simulink model "LoadFlow58BusNetwork_2024"  (R2024a)
settings: Solver=FixedStepDiscrete  StartTime=0.0  StopTime=4.5  FixedStep=75e-6  RelTol=1e-3  EnableMultiTasking=on
undefined symbols (not defined in the file): D1, D11, Delta
libraries: spsSeriesRLCBranchLib x41, spsLoadFlowBusLib x29, spsDistributedParametersLineLib x19, spsThreePhaseSeriesRLCLoadLib x15, spsThreePhaseTransformerTwoWindingsLib x13, spsThreePhaseParallelRLCLoadLib x11, spsThreePhaseVIMeasurementLib x11, spsSynchronousMachinepuStandardLib x7, spsExcitationSystemLib x7, spsHydraulicTurbineandGovernorLib x7, spsGenericPowerSystemStabilizerLib x7, spsMultiBandPowerSystemStabilizerLib x7
(part 1 of 5)
settings Model: Creator=The MathWorks, Inc.  LastModifiedBy=dilu2
settings SolverCC: AlgebraicLoopSolver=TrustRegion
settings DataIOCC: SaveFormat=StructureWithTime  SaveOutput=off  SaveTime=off  ReturnWorkspaceOutputs=off
settings OptimizationCC: ExpressionDepthLimit=2147483647  LifeSpan=inf
settings DebuggingCC: UnderspecifiedInitializationDetection=Classic  MergeDetectMultiDrivingBlocksExec=none  SolverPrmCheckMsg=warning  FcnCallInpInsideContextMsg=warning  UnconnectedInputMsg=warning  UnconnectedOutputMsg=warning  UnconnectedLineMsg=warning  StateNameClashWarn=warning  SFUnexpectedBacktrackingDiag=warning  SFNoUnconditionalDefaultTransitionDiag=warning  SFExecutionAtInitializationDiag=none  ArithmeticOperatorsInVariantConditions=warning
settings HardwareCC: ProdBitPerPointer=32  ProdBitPerSizeT=32  ProdBitPerPtrDiffT=32  ProdLargestAtomicFloat=None  ProdIntDivRoundTo=Undefined  ProdEndianess=Unspecified  ProdWordSize=32  ProdHWDeviceType=32-bit Generic
settings ModelReferenceCC: EnableRefExpFcnMdlSchedulingChecks=on  PropagateSignalLabelsOutOfModel=off
settings SFSimCC: SimUseLocalCustomCode=off  CustomCodeUndefinedFunction=UseInterfaceOnly
settings RTWCC: RTWUseLocalCustomCode=off  GPUComputeCapability=3.5
settings CodeAppCC: StateflowObjectComments=on
settings GRTTargetCC: TargetLangStandard=C89/C90 (ANSI)  CombineOutputUpdateFcns=off  GRTInterface=on
settings ConfigComp: CovMetricSettings=dw  CovSaveCumulativeToWorkspaceVar=on  CovSaveSingleToWorkspaceVar=on  CovExternalEMLEnable=off  CovSFcnEnable=off
settings SimscapeCC: SimscapeNormalizeSystem=off

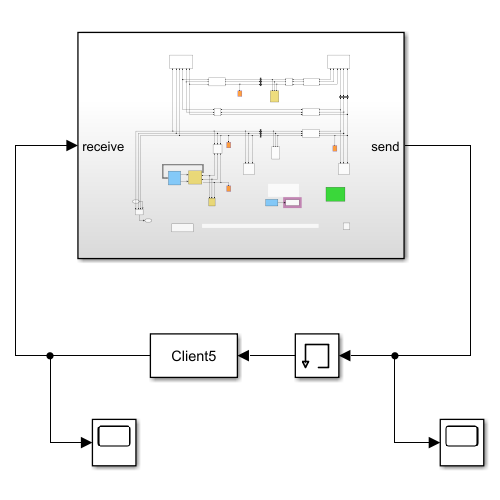
[thumbnail: Simulink's stored preview of the top-level diagram]
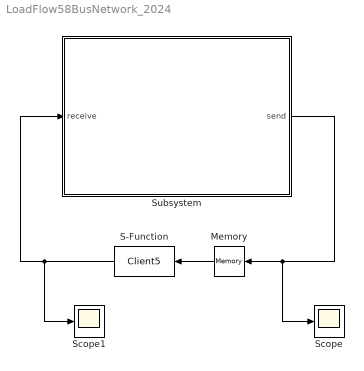
== system LoadFlow58BusNetwork_2024 ==
  Memory : Memory
  S-Function : S-Function  FunctionName=Client5  SFunctionDeploymentMode=off  EnableBusSupport=off
  Scope : Scope
  Scope1 : Scope
  Subsystem : Subsystem
  wires:
  Memory/1 -> S-Function/1
  Subsystem/1(send) -> Scope/1, Memory/1
  S-Function/1 -> Scope1/1, Subsystem/1(receive)

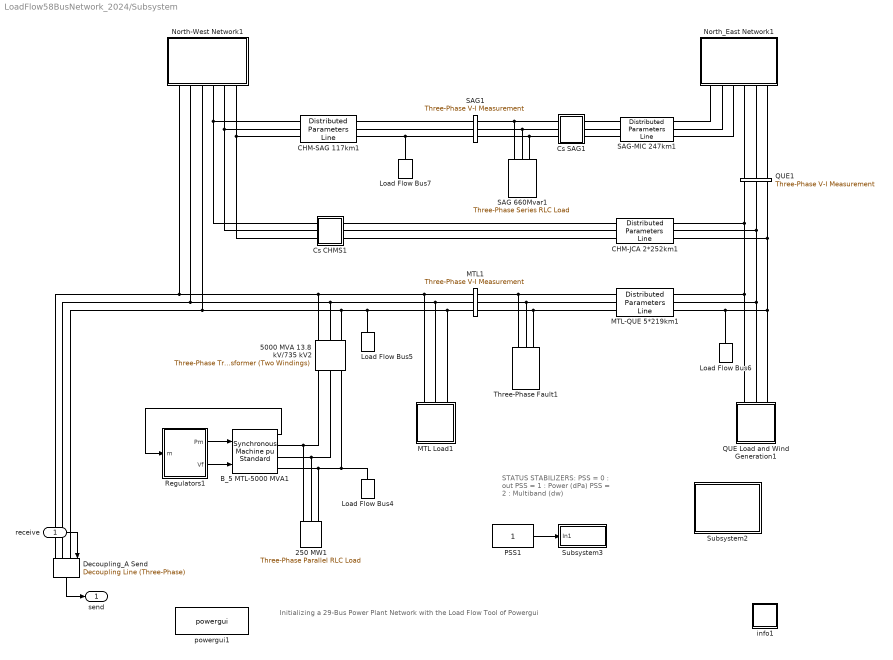
== system LoadFlow58BusNetwork_2024/Subsystem ==
  note: Initializing a 29-Bus Power Plant Network with the Load Flow Tool of Powergui
  note: STATUS STABILIZERS:
      | PSS = 0 :  out
      | PSS = 1 :  Power (dPa)
      | PSS = 2 :  Multiband (dw)
  receive : Inport
  250 MW1 : spsThreePhaseParallelRLCLoadLib/Three-Phase Parallel RLC Load  LConnTagsString=A|B|C  Configuration=Y (grounded)  NominalVoltage=(13800)*1  Vabc=[1e3 1e3 1e3]  Vabcp=[1e3 1e3 1e3]  NominalFrequency=60  UnbalancedPower=off  ActivePower=250000000  InductivePower=0  CapacitivePower=0  Pabc=[10e3 9e3 11e3]  QLabc=[100 90 110]  QCabc=[100 90 110]  Pabcp=[10e3 9e3 11e3]  QLabcp=[100 90 110]  QCabcp=[100 90 110]  Measurements=None  LoadType=constant PQ
  5000 MVA 13.8 kV/735 kV2 : spsThreePhaseTransformerTwoWindingsLib/Three-Phase Transformer (Two Windings)  Winding1Connection=Delta (D1)  Winding2Connection=Yg  CoreType=Three single-phase transformers  SetSaturation=off  Hysteresis=off  DataFile='basic_model'  SetInitialFlux=off  Measurements=None  UNITS=pu  NominalPower=[ 5000e6 60 ]  Winding1="[ 13.8e3 0.002  0.0]"  Winding2=[ 735e3 0.002 0.12]  Rm=500  Lm=500  L0=0.5  Saturation="[ 0,0  ;  0.005,1.2  ;  1.0,1.4 ]"  InitialFluxes=[ 0.8 , -0.8 , 0.7 ]  BreakLoop=off  DiscreteSolver=Trapezoidal iterative  DataType=off  TransfoNumber=0
  B_5 MTL-5000 MVA1 : spsSynchronousMachinepuStandardLib/Synchronous Machine pu Standard  PresetModel=No  MechanicalLoad=Mechanical power Pm  ShowDetailedParameters=on  RotorType=Salient-pole  Units=per unit standard parameters  MeasurementBus=off  NominalParameters="[5000E6  13800   60 ]"  Reactances1=[ 31 32 33 34 35 36 37 ]  Reactances2=[ 1.305, 0.296, 0.252, 0.474, 0.243, 0.18 ]  dAxisTimeConstants=Short-circuit  qAxisTimeConstants=Open-circuit  TimeConstants1=[]  TimeConstants2=[]  TimeConstants3=[]  TimeConstants4=[]  TimeConstants5=[ 1.01, 0.053, 0.1 ]  TimeConstants6=[]  TimeConstants7=[]  TimeConstants8=[]  StatorResistance=2.8544e-3  Mechanical="[ 3.7 0  32]"  PolePairs=32  InitialConditions=[0 -113.876 0.904539 0.904539 0.904539 -42.1129 -162.113 77.8871 1.28555]  SetSaturation=off  Saturation=[0.6404,0.7127,0.8441,0.9214,0.9956,1.082,1.19,1.316,1.457;0.7,0.7698,0.8872,0.9466,0.9969,1.046,1.1,1.151,1.201]  LoadFlowParameters=[1 4000000000 0 0 0]  TsPowergui=0  TsBlock=-1  IterativeModel=Trapezoidal non iterative  IterativeDiscreteModel=Trapezoidal non iterative  BusType=PV  Pref=4500000000  Qref=0  Qmin=-Inf  Qmax=Inf  PLF=0  QLF=0
  CHM-JCA 2*252km1 : spsDistributedParametersLineLib/Distributed Parameters Line  Phases=3  Length=252  Frequency=60  Resistance="[0.01273  0.3864]/2"  Inductance="[0.9337e-3  4.1264e-3]/2"  Capacitance=[12.74e-9 7.751e-9]*2  x1=[-0.0015 2.08314728731826e-08 15714.262594831 -742648.807936676;-0.001425 2.08441228975103e-08 36703.0761534446 -741907.711972178;-0.00135 2.08401104489196e-08 57662.549834557 -740573.546334299;-0.001275 2.08194387349004e-08 78575.9289555982 -738647.377534635;-0.0012 2.07821242801046e-08 99426.4956812844 -736130.745323054;-0.001125 2.07281969131365e-08 120197.582387599 -733025.66145684;-0.00105 2.0657699742708e-08 140872.584985638 -729334.608092525;-0.000975 2.05706891231786e-08 161434.976194663 -725060.535801696;-0.0009 2.04672346095063e-08 181868.318753755 -720206.861212344;-0.000825 2.03474189016463e-08 202156.278561514 -714777.464277674;-0.00075 2.02113377784423e-08 222282.637733286 -708776.685174523;-0.000675 2.0059100021062e-08 242231.307565492 -702209.32083389;-0.0006 1.98908273260395e-08 261986.341396694 -695080.621106345;-0.000525 1.97066542079923e-08 281531.947355108 -687396.284565378;-0.00045 1.95067278920932e-08 300852.50098239 -679162.453952045;-0.000375 1.92912081963801e-08 319932.557723585 -670385.711264557;-0.0003 1.90602674040002e-08 338756.865273267 -661073.072496729;-0.000225 1.88140901254894e-08 357310.375768004 -651231.982029504;-0.00015 1.85528731511975e-08 375578.257815384 -640870.306680029;-7.5e-05 1.82768252939771e-08 393545.908350007 -629996.329413038]  x2=[-0.0015 1.40076837789875e-08 -209700.603633346 -700128.672634885;-0.001425 1.39707979514796e-08 -189823.746323601 -705777.196573694;-0.00135 1.39227440818497e-08 -169795.146815445 -710861.533020316;-0.001275 1.38635605836259e-08 -149630.815664878 -715377.617633987;-0.0012 1.37932947671911e-08 -129346.871929697 -719321.840325766;-0.001125 1.37120028019639e-08 -108959.530284169 -722691.048144382;-0.00105 1.36197496714975e-08 -88485.0880572684 -725482.547796656;-0.000975 1.35166091215329e-08 -67939.9122048419 -727694.107800476;-0.0009 1.34026636010476e-08 -47340.4262261144 -729323.960268613;-0.000825 1.32780041963472e-08 -26703.0970349947 -730370.802321943;-0.00075 1.31427305582526e-08 -6044.42179667621 -730833.797130944;-0.000675 1.29969508224402e-08 14619.0852599438 -730712.574584651;-0.0006 1.28407815230003e-08 35270.9060434865 -730007.231586512;-0.000525 1.26743474992815e-08 55894.531804401 -728718.331976929;-0.00045 1.24977817960958e-08 76473.4763318061 -726846.906082527;-0.000375 1.23112255573648e-08 96991.2891323149 -724394.449892533;-0.0003 1.21148279132913e-08 117431.568580308 -721362.923862902;-0.000225 1.1908745861147e-08 137777.975029141 -717754.751349158;-0.00015 1.16931441397712e-08 158014.24387281 -713572.816669202;-7.5e-05 1.14681950978812e-08 178124.198547625 -708820.46279763]  x3=[-0.0015 5.29913482848101e-11 0.894999888004861 -284.908126309882;-0.001425 5.24485107921031e-11 8.94952227191277 -284.768519995041;-0.00135 5.18637467623581e-11 16.9968905446488 -284.40127408242;-0.001275 5.12375236469932e-11 25.0306717631445 -283.806682142784;-0.0012 5.05703420391853e-11 33.0444438456149 -282.98521948383;-0.001125 4.98627352737034e-11 41.0318007052721 -281.937542770241;-0.00105 4.91152690005692e-11 48.9863573712531 -280.664489498749;-0.000975 4.83285407328847e-11 56.901755092668 -279.167077328663;-0.0009 4.75031793691899e-11 64.7716664216877 -277.44650326836;-0.000825 4.66398446907303e-11 72.5898002716097 -275.504142718419;-0.00075 4.57392268340385e-11 80.3499069458558 -273.341548372142;-0.000675 4.48020457392492e-11 88.0457831338842 -270.960448974363;-0.0006 4.38290505745903e-11 95.6712768700209 -268.362747939508;-0.000525 4.2821019137509e-11 103.220292451247 -265.550521830038;-0.00045 4.17787572329127e-11 110.686795310012 -262.526018696476;-0.000375 4.07030980290208e-11 118.06481683817 -259.291656280351;-0.0003 3.95949013913429e-11 125.3484591582 -255.850020081491;-0.000225 3.8455053195315e-11 132.531899837875 -252.203861291214;-0.00015 3.72844646181448e-11 139.609396544626 -248.356094593069;-7.5e-05 3.60840714104303e-11 146.575291635874 -244.309795832883]  x4=[-0.0015 3.38337818505227e-11 -3172.8334199357 -10043.3125795465;-0.001425 3.4961387413953e-11 -2887.63550825271 -10128.9965094924;-0.00135 3.60610453792117e-11 -2600.12926492673 -10206.5834746075;-0.001275 3.71318766965467e-11 -2310.54451804968 -10276.011453059;-0.0012 3.81730253597873e-11 -2019.11275723742 -10337.2249451831;-0.001125 3.91836590906222e-11 -1726.06694858048 -10390.1750178508;-0.00105 4.01629700039101e-11 -1431.64134841455 -10434.8193435843;-0.000975 4.1110175253491e-11 -1136.07131605956 -10471.1222343927;-0.0009 4.20245176579809e-11 -839.593125676973 -10499.0546703004;-0.000825 4.29052663060518e-11 -542.44377739593 -10518.5943225456;-0.00075 4.37517171407102e-11 -244.860807858905 -10529.7255714292;-0.000675 4.456319352211e-11 52.9178996614269 -10532.4395188013;-0.0006 4.5339046768448e-11 350.65430542244 -10526.7339951737;-0.000525 4.607865667451e-11 648.110403496889 -10512.6135614548;-0.00045 4.67814320074534e-11 945.048412031206 -10490.0895053033;-0.000375 4.744681097943e-11 1241.23096332467 -10459.179832105;-0.0003 4.80742616966702e-11 1536.42129357752 -10419.9092505798;-0.000225 4.86632825846709e-11 1830.38343215632 -10372.3091530295;-0.00015 4.92134027891467e-11 2122.88239022526 -10316.417590244;-7.5e-05 4.97241825524231e-11 2413.68434859265 -10252.2792410834]  x5=0.00142516474882927  V1=ones(3,3)  V2=ones(3,3)  I1=ones(3,3)  I2=ones(3,3)  nHarmo=1  Measurements=None  Decoupling=on  VsMag0=[606505.937088385 606505.59619374 606505.952336152]  VrMag0=[596743.737336323 596743.911083336 596743.706580344]  VsAngle0=[3.61218308623149 -116.387796657602 123.612221103661]  VrAngle0=[-14.273856882167 -134.273869923453 105.726122150021]  IsMag0=[234.023435046632 234.012623108715 234.010085805107]  IrMag0=[8650.9003206612 8650.90619032986 8650.91364627862]  IsAngle0=[2.58186505632488 -117.420380634369 122.583034804954]  IrAngle0=[-15.1321830152099 -135.132103549669 104.867823050539]
      settings: AttributesFormatString=\n  LibrarySourceBlock=sps_lib/Power Grid Elements/Distributed Parameters Line
  CHM-SAG 117km1 : spsDistributedParametersLineLib/Distributed Parameters Line  Phases=3  Length=117  Frequency=60  Resistance="[0.01273  0.3864]"  Inductance="[0.9337e-3  4.1264e-3]"  Capacitance=[12.74e-9 7.751e-9]  x1=[-0.000675 1.91802413039641e-08 161384.253868462 -730188.013921057;-0.0006 1.90228604750691e-08 181962.578167363 -725333.731757154;-0.000525 1.88502730625698e-08 202395.444365398 -719899.628906063;-0.00045 1.86626170302032e-08 222666.518741962 -713890.049306458;-0.000375 1.84600423873302e-08 242759.596910355 -707309.796924322;-0.0003 1.82427110690209e-08 262658.616771325 -700164.131912727;-0.000225 1.80107968066059e-08 282347.671352859 -692458.766406951;-0.00015 1.77644849887981e-08 301811.021525978 -684199.859958284;-7.5e-05 1.7503972513496e-08 321033.108586353 -675394.014610176]  x2=[-0.000675 1.32644576582055e-08 211241.020698699 -709610.354234679;-0.0006 1.31314025060213e-08 231217.678579178 -703354.834381429;-0.000525 1.29878503115909e-08 251009.504585149 -696537.063435265;-0.00045 1.28339158283422e-08 270600.67743373 -689162.491417966;-0.000375 1.26697221091458e-08 289975.536241099 -681237.013449566;-0.0003 1.24954004079486e-08 309118.593041571 -672766.965035891;-0.000225 1.23110900748514e-08 328014.54516844 -663759.117004046;-0.00015 1.21169384447143e-08 346648.287486691 -654220.670089923;-7.5e-05 1.19131007193799e-08 365004.924467822 -644159.249182042]  x3=[-0.000675 1.53791884966281e-11 931.801693491258 -3923.77003572315;-0.0006 1.43946793528256e-11 1042.35686429523 -3895.85908672161;-0.000525 1.33986633225944e-11 1152.07879097047 -3864.83384757478;-0.00045 1.23919366059096e-11 1260.87976348761 -3830.71911938414;-0.000375 1.1375303964705e-11 1368.67280801392 -3793.54217294144;-0.0003 1.0349578079559e-11 1475.37175643891 -3753.33272692882;-0.000225 9.31557890005e-12 1580.89131525574 -3710.12292416222;-0.00015 8.27413298930147e-12 1685.14713374361 -3663.94730589682;-7.5e-05 7.22607286323979e-12 1788.05587139637 -3614.84278421537]  x4=[-0.000675 2.92162426308819e-11 34.7429415929704 -1477.32347167481;-0.0006 2.99900814486756e-11 76.4934319414226 -1475.75088744197;-0.000525 3.07399466542229e-11 118.18277461077 -1472.99861052946;-0.00045 3.14652388167517e-11 159.77764377835 -1469.06884106533;-0.000375 3.21653781488047e-11 201.244789142174 -1463.96472044716;-0.0003 3.28398049697123e-11 242.551062500706 -1457.69032883087;-0.000225 3.34879801529931e-11 283.663444251031 -1450.25068186913;-0.00015 3.41093855573228e-11 324.549069784217 -1441.65172670188;-7.5e-05 3.4703524440729e-11 365.175255756786 -1431.90033720231]  x5=0.000661683633385019  V1=ones(3,3)  V2=ones(3,3)  I1=ones(3,3)  I2=ones(3,3)  nHarmo=1  Measurements=None  Decoupling=on  VsMag0=[610584.183721716 610584.009535667 610584.14443005]  VrMag0=[604521.569069134 604521.776249714 604521.565003261]  VsAngle0=[-2.95698942544824 -122.956984245967 117.043027319659]  VrAngle0=[1.15752648646476 -118.842485295541 121.157503589918]  IsMag0=[3301.92473587884 3301.9203040404 3301.91445622792]  IrMag0=[1209.87683704248 1209.87940955586 1209.88665322207]  IsAngle0=[-2.06102029188923 -122.061181862043 117.93896552265]  IrAngle0=[-14.0730509971364 -134.07258455703 105.92707671982]
      settings: AttributesFormatString=\n  LibrarySourceBlock=sps_lib/Power Grid Elements/Distributed Parameters Line
  Cs CHMS1 : Subsystem  mask{Xc=33/2}
      mask prompts: Xc "Condensator Reactance at  60Hz  (ohm):"
      mask help: Series Compensation
      mask init:
      | Cs=1/Xc/(2*pi*60);
      mask Display: disp('Cs')
  Cs SAG1 : Subsystem  mask{Xc=22}
      mask prompts: Xc "Condensator Reactance at  60Hz  (ohm):"
      mask help: Series Compensation
      mask init:
      | Cs=1/Xc/(2*pi*60);
      mask Display: disp('Cs')
  Decoupling_A Send : spsDecouplingLineThreePhaseLib/Decoupling Line (Three-Phase)  Length=252  Frequency=60  Resistance="[0.01273  0.3864]/2"  Inductance="[0.9337e-3  4.1264e-3]/2"  Capacitance=[12.74e-9 7.751e-9]*2  VsMag0=[520613.013363934 520613.032750504 520613.042981031]  VsAngle0=[95.9069967092205 -144.093005822696 -24.0930027089948]  IhsMag0=[3886.83215054359 3886.83229528369 3886.83237166141]  IhsAngle0=[86.4922430478757 -153.50775948403 -33.5077563702981]  ShowPorts=on  ConnectorID=T34_3229_1960624034510_S
      settings: LibrarySourceBlock=|
      | sps_lib/Power Grid Elements/Decoupling Line
      | (Three-Phase)
  Load Flow Bus4 : spsLoadFlowBusLib/Load Flow Bus  LConnTagsString=a  Phases=single  Connectors=on one side  ID=MTL_13.8  Vbase=13.8e3  Vref=1  Vangle=0  VLF=1  VLFb=1  VLFc=1  angleLF=-47.86  angleLFb=0  angleLFc=0
      settings: AttributesFormatString=%<ID>\n%<Vbase>V\n%<VLF>pu\n%<angleLF>deg.
  Load Flow Bus5 : spsLoadFlowBusLib/Load Flow Bus  LConnTagsString=a  Phases=single  Connectors=on one side  ID=MTL7  Vbase=735e3  Vref=1  Vangle=0  VLF=1.013  VLFb=1  VLFc=1  angleLF=-23.64  angleLFb=0  angleLFc=0
      settings: AttributesFormatString=%<ID>\n%<Vbase>V\n%<VLF>pu\n%<angleLF>deg.
  Load Flow Bus6 : spsLoadFlowBusLib/Load Flow Bus  LConnTagsString=a  Phases=single  Connectors=on one side  ID=QUE7  Vbase=735e3  Vref=1  Vangle=0  VLF=1.023  VLFb=1  VLFc=1  angleLF=-14.99  angleLFb=0  angleLFc=0
      settings: AttributesFormatString=%<ID>\n%<Vbase>V\n%<VLF>pu\n%<angleLF>deg.
  Load Flow Bus7 : spsLoadFlowBusLib/Load Flow Bus  LConnTagsString=a  Phases=single  Connectors=on one side  ID=SAG7  Vbase=735e3  Vref=1  Vangle=0  VLF=1.036  VLFb=1  VLFc=1  angleLF=-0.1653  angleLFb=0  angleLFc=0
      settings: AttributesFormatString=%<ID>\n%<Vbase>V\n%<VLF>pu\n%<angleLF>deg.
  MTL Load1 : Subsystem
  MTL-QUE 5*219km1 : spsDistributedParametersLineLib/Distributed Parameters Line  Phases=3  Length=219  Frequency=60  Resistance="[0.01273  0.3864]/5"  Inductance="[0.9337e-3  4.1264e-3]/5"  Capacitance=[12.74e-9 7.751e-9]*5  x1=[-0.001275 8.74149343994407e-08 0 0;-0.0012 8.73707129290097e-08 0 0;-0.001125 8.72566486474799e-08 0 0;-0.00105 8.70728327360928e-08 0 0;-0.000975 8.68194121344755e-08 0 0;-0.0009 8.64965894231794e-08 0 0;-0.000825 8.61046226617407e-08 -143097.879675133 -713663.77653503;-0.00075 8.56438251823911e-08 -122864.998636676 -717423.987747158;-0.000675 8.51145653395851e-08 -102533.901198206 -720610.701200436;-0.0006 8.45172662155432e-08 -82120.8397279397 -723221.369484888;-0.000525 8.38524052820461e-08 -61642.1321148858 -725253.905672232;-0.00045 8.31205140187514e-08 -41114.1487245756 -726706.684984138;-0.000375 8.23221774883366e-08 -20553.2993128425 -727578.546091053;-0.0003 8.14580338688091e-08 23.980091885227 -727868.792040548;-0.000225 8.05287739433567e-08 20601.2403272944 -727577.190814451;-0.00015 7.95351405481455e-08 41162.0322463955 -726703.975514322;-7.5e-05 7.84779279785086e-08 61689.9198667191 -725249.844175111]  x2=[-0.001275 1.38635605836259e-08 0 0;-0.0012 1.37932947671911e-08 0 0;-0.001125 1.37120028019639e-08 0 0;-0.00105 1.36197496714975e-08 0 0;-0.000975 1.35166091215329e-08 0 0;-0.0009 1.34026636010476e-08 0 0;-0.000825 1.32780041963472e-08 -26703.0970349947 -730370.802321943;-0.00075 1.31427305582526e-08 -6044.42179667621 -730833.797130944;-0.000675 1.29969508224402e-08 14619.0852599438 -730712.574584651;-0.0006 1.28407815230003e-08 35270.9060434865 -730007.231586512;-0.000525 1.26743474992815e-08 55894.531804401 -728718.331976929;-0.00045 1.24977817960958e-08 76473.4763318061 -726846.906082527;-0.000375 1.23112255573648e-08 96991.2891323149 -724394.449892533;-0.0003 1.21148279132913e-08 117431.568580308 -721362.923862902;-0.000225 1.1908745861147e-08 137777.975029141 -717754.751349158;-0.00015 1.16931441397712e-08 158014.24387281 -713572.816669202;-7.5e-05 1.14681950978812e-08 178124.198547625 -708820.46279763]  x3=[-0.001275 3.38356403910686e-10 0 0;-0.0012 3.13475237189635e-10 0 0;-0.001125 2.88343483160307e-10 0 0;-0.00105 2.62981231762344e-10 0 0;-0.000975 2.37408757191458e-10 0 0;-0.0009 2.11646501692549e-10 0 0;-0.000825 1.85715059218486e-10 -5323.24056616569 -20344.1866352303;-0.00075 1.59635158967621e-10 -4745.97060123439 -20486.5462812051;-0.000675 1.33427648813176e-10 -4164.90678002025 -20612.5292955374;-0.0006 1.07113478637782e-10 -3580.51359605137 -20722.0349693331;-0.000525 8.07136835864552e-11 -2993.2582042975 -20814.9757654321;-0.00045 5.42493672514307e-11 -2403.6100477335 -20891.277388384;-0.000375 2.77416848022685e-11 -1812.04048207381 -20950.8788438389;-0.0003 1.21182607473737e-12 -1219.0223989779 -20993.7324873053;-0.000225 -2.53190013680163e-11 -625.029848027918 -21019.8040622361;-0.00015 -5.18295891884701e-11 -30.5376577806965 -21029.0727274134;-7.5e-05 -7.8298745228346e-11 563.978943802912 -21021.531073608]  x4=[-0.001275 2.95644055162341e-10 0 0;-0.0012 3.24049227246394e-10 0 0;-0.001125 3.52195359336306e-10 0 0;-0.00105 3.80059951844735e-10 0 0;-0.000975 4.07620730242771e-10 0 0;-0.0009 4.34855662865857e-10 0 0;-0.000825 4.61742978525563e-10 -1592.00824148551 -5672.40977476208;-0.00075 4.8826118391314e-10 -1431.01007071774 -5715.14957068699;-0.000675 5.14389080780944e-10 -1268.86797239464 -5753.32076348981;-0.0006 5.40105782887988e-10 -1105.71156042873 -5786.89283970306;-0.000525 5.65390732696087e-10 -941.671259559369 -5815.83896232268;-0.00045 5.90223717803237e-10 -776.878201093171 -5840.13599226114;-0.000375 6.14584887101101e-10 -611.464118079654 -5859.76450684446;-0.0003 6.3845476664368e-10 -445.561240005859 -5874.70881533841;-0.000225 6.6181427521449e-10 -279.302187094119 -5884.95697149145;-0.00015 6.84644739579792e-10 -112.819864287482 -5890.50078308433;-7.5e-05 7.06927909415689e-10 53.752644992464 -5891.3358184789]  x5=0.00123853603172068  V1=ones(3,3)  V2=ones(3,3)  I1=ones(3,3)  I2=ones(3,3)  nHarmo=1  Measurements=None  Decoupling=on  VsMag0=[594302.518281079 594302.525591473 594302.380387402]  VrMag0=[596743.737336323 596743.911083336 596743.706580344]  VsAngle0=[-23.5181046799965 -143.51812043764 96.4818868308265]  VrAngle0=[-14.273856882167 -134.273869923453 105.726122150021]  IsMag0=[17258.8321886677 17258.8369567323 17258.821705247]  IrMag0=[4835.28137561733 4835.27973459469 4835.28879561644]  IsAngle0=[-26.8431826212202 -146.843231946901 93.1567790076211]  IrAngle0=[-27.8572964468753 -147.857183694816 92.1427767692567]
      settings: AttributesFormatString=\n  LibrarySourceBlock=sps_lib/Power Grid Elements/Distributed Parameters Line
  MTL1 : spsThreePhaseVIMeasurementLib/Three-Phase V-I Measurement  VoltageMeasurement=phase-to-ground  SetLabelV=on  LabelV=Vabc_MTL7_1  Vpu=on  VpuLL=off  CurrentMeasurement=no  SetLabelI=off  LabelI=A1  Ipu=off  Pbase=100e6  Vbase=735e3  OutputType=Magnitude  PhasorSimulation=off  PSBequivalent=0
  North-West Network1 : Subsystem
  North_East Network1 : Subsystem
  PSS1 : Constant
  QUE Load and Wind Generation1 : Subsystem
  QUE1 : spsThreePhaseVIMeasurementLib/Three-Phase V-I Measurement  VoltageMeasurement=no  SetLabelV=on  LabelV=Vabc_QUE7  Vpu=on  VpuLL=off  CurrentMeasurement=no  SetLabelI=off  LabelI=A1  Ipu=off  Pbase=100e6  Vbase=735e3  OutputType=Magnitude  PhasorSimulation=off  PSBequivalent=0
  Regulators1 : Subsystem
  SAG 660Mvar1 : spsThreePhaseSeriesRLCLoadLib/Three-Phase Series RLC Load  LConnTagsString=A|B|C  Configuration=Y (grounded)  NominalVoltage=735e3  Vabc=[1e3 1e3 1e3]  Vabcp=[1e3 1e3 1e3]  NominalFrequency=60  UnbalancedPower=off  ActivePower=2200000  InductivePower=660e6  CapacitivePower=0  Pabc=[10e3 9e3 11e3]  QLabc=[100 90 110]  QCabc=[100 90 110]  Pabcp=[10e3 9e3 11e3]  QLabcp=[100 90 110]  QCabcp=[100 90 110]  Measurements=None  LoadType=constant Z
  SAG-MIC 247km1 : spsDistributedParametersLineLib/Distributed Parameters Line  Phases=3  Length=247  Frequency=60  Resistance="[0.01273  0.3864]/1"  Inductance="[0.9337e-3  4.1264e-3]/1"  Capacitance=[12.74e-9 7.751e-9]*1  x1=[-0.001425 1.47124469074144e-08 -23892.3616667774 -729222.084147013;-0.00135 1.46899929834646e-08 -3267.28940140246 -729606.070163554;-0.001275 1.46557961038881e-08 17360.3946851287 -729406.820250953;-0.0012 1.46098836051474e-08 37974.2011377716 -728624.493686542;-0.001125 1.45522921889915e-08 58557.6515950497 -727259.715850207;-0.00105 1.44830678931173e-08 79094.2919616048 -725313.577724468;-0.000975 1.44022660543676e-08 99567.7055613491 -722787.635022366;-0.0009 1.43099512644962e-08 119961.526260705 -719683.906943849;-0.000825 1.42061973185335e-08 140259.45155144 -716004.874561653;-0.00075 1.40910871557964e-08 160445.255582647 -711753.478837975;-0.000675 1.39647127935879e-08 180502.802131436 -706933.118273508;-0.0006 1.38271752536395e-08 200416.057501987 -701547.646190732;-0.000525 1.36785844813562e-08 220169.103342639 -695601.36765363;-0.00045 1.35190592579279e-08 239746.149370779 -689099.036026284;-0.000375 1.33487271053773e-08 259131.545995351 -682045.849173106;-0.0003 1.3167724184621e-08 278309.7968269 -674447.445303752;-0.000225 1.29761951866245e-08 297265.571065148 -666309.898466013;-0.00015 1.27742932167383e-08 315983.715754203 -657639.713690325;-7.5e-05 1.25621796723078e-08 334449.267895597 -648443.821789737]  x2=[-0.001425 4.75263384881545e-09 88893.3544414114 -739233.912944179;-0.00135 4.71488557756924e-09 109756.40330771 -736425.413361934;-0.001275 4.67336829893249e-09 130531.714584533 -733028.226571933;-0.0012 4.62811520118251e-09 151202.68080592 -729045.068233319;-0.001125 4.57916245895323e-09 171752.777917749 -724479.122421923;-0.00105 4.52654920431781e-09 192165.578486817 -719334.039084965;-0.000975 4.47031749550698e-09 212424.764832674 -713613.931123342;-0.0009 4.41051228328839e-09 232514.142071731 -707323.371103838;-0.000825 4.34718137503364e-09 252417.651063202 -700467.387603885;-0.00075 4.2803753965018e-09 272119.381246533 -693051.461191792;-0.000675 4.21014775136993e-09 291603.583360062 -685081.520045664;-0.0006 4.13655457854304e-09 310854.682030736 -676563.935214511;-0.000525 4.05965470727746e-09 329857.288224832 -667505.515525323;-0.00045 3.97950961015369e-09 348596.211549706 -657913.502140201;-0.000375 3.8961833539361e-09 367056.472396769 -647795.562767882;-0.0003 3.80974254835898e-09 385223.31391595 -637159.785534291;-0.000225 3.72025629287972e-09 403082.213812101 -626014.672517016;-0.00015 3.62779612144176e-09 420618.895953895 -614369.132948876;-7.5e-05 3.53243594529146e-09 437819.341785948 -602232.476096019]  x3=[-0.001425 1.449181420039e-11 -591.222973545874 -3970.47337116317;-0.00135 1.3927631720128e-11 -478.738749485206 -3985.6004368759;-0.001275 1.33523157041689e-11 -365.871828993148 -3997.54147458112;-0.0012 1.27663260513332e-11 -252.71243615902 -4006.28693879599;-0.001125 1.21701311927833e-11 -139.351028870057 -4011.82983853024;-0.00105 1.15642077175673e-11 -25.8782265007565 -4014.16574287462;-0.000975 1.09490399916401e-11 87.6152625268583 -4013.29278454294;-0.0009 1.03251197706695e-11 201.038713254167 -4009.21166136473;-0.000825 9.69294580693383e-12 314.301456710097 -4001.92563572743;-0.00075 9.05302345062717e-12 427.312952390505 -3991.44053196844;-0.000675 8.40586424588999e-12 539.982860634881 -3977.76473171929;-0.0006 7.75198552188868e-12 652.221114842479 -3960.90916720544;-0.000525 7.09190997927053e-12 763.93799347019 -3940.88731250727;-0.00045 6.42616527232481e-12 875.044191754565 -3917.71517278907;-0.000375 5.75528358718402e-12 985.450893100676 -3891.41127150481;-0.0003 5.07980121640243e-12 1095.06984008075 -3861.99663559069;-0.000225 4.40025813025201e-12 1203.81340498579 -3829.49477865661;-0.00015 3.71719754507847e-12 1311.59465987384 -3793.9316821897;-7.5e-05 3.03116548906243e-12 1418.32744605887 -3755.33577478516]  x4=[-0.001425 9.72811966664692e-12 -44.2696955264446 -1445.03567527927;-0.00135 1.03978814794709e-11 -3.40032222034586 -1445.70991618316;-0.001275 1.10593313849332e-11 37.471769251309 -1445.22847870017;-0.0012 1.17119406300998e-11 78.3139063639618 -1443.59174768403;-0.001125 1.23551875291253e-11 119.09344053811 -1440.8010315125;-0.00105 1.29885578802808e-11 159.777773238083 -1436.85856104137;-0.000975 1.36115453769985e-11 200.334382030812 -1431.76748782121;-0.0009 1.42236520126053e-11 240.730846583763 -1425.53188157807;-0.000825 1.48243884784225e-11 280.934874581261 -1418.15672696016;-0.00075 1.54132745549107e-11 320.914327538467 -1409.64791955325;-0.000675 1.59898394955508e-11 360.637246492392 -1400.01226116778;-0.0006 1.65536224031509e-11 400.071877549406 -1389.25745440164;-0.000525 1.71041725982808e-11 439.186697268812 -1377.3920964828;-0.00045 1.76410499795383e-11 477.950437862204 -1364.42567239684;-0.000375 1.81638253753592e-11 516.332112188455 -1350.36854730478;-0.0003 1.86720808870909e-11 554.301038524369 -1335.23195825734;-0.000225 1.91654102230539e-11 591.826865091176 -1319.0280052122;-0.00015 1.96434190233252e-11 628.879594317285 -1301.7696413615;-7.5e-05 2.01057251749837e-11 665.429606817877 -1283.47066277723]  x5=0.00139688767047948  V1=ones(3,3)  V2=ones(3,3)  I1=ones(3,3)  I2=ones(3,3)  nHarmo=1  Measurements=None  Decoupling=on  VsMag0=[595726.858585737 595726.856922626 595726.834929731]  VrMag0=[607930.23167611 607930.976808519 607930.152146887]  VsAngle0=[-1.09657636564089 -121.096578900452 118.903422505478]  VrAngle0=[7.63692875074935 -112.363120449623 127.636843332422]  IsMag0=[3296.72064632886 3296.71771518503 3296.71033953548]  IrMag0=[1187.28543067559 1187.29227239663 1187.29553954474]  IsAngle0=[-7.68926033426767 -127.689437762273 112.310695069139]  IrAngle0=[-0.975042579703497 -120.974669903312 119.024857828983]
      settings: AttributesFormatString=\n  LibrarySourceBlock=sps_lib/Power Grid Elements/Distributed Parameters Line
  SAG1 : spsThreePhaseVIMeasurementLib/Three-Phase V-I Measurement  VoltageMeasurement=no  SetLabelV=on  LabelV=Vabc_SAG7  Vpu=on  VpuLL=off  CurrentMeasurement=no  SetLabelI=off  LabelI=Iabc_SAG7  Ipu=off  Pbase=100e6  Vbase=735e3  OutputType=Magnitude  PhasorSimulation=off  PSBequivalent=0
  Subsystem2 : Subsystem
      mask Display: disp('Display\nWaveforms')
  Subsystem3 : Subsystem
      mask Display: disp('PSS_select')
  Three-Phase Fault1 : spsThreePhaseFaultLib/Three-Phase Fault  InitialStates=0  FaultA=on  FaultB=on  FaultC=on  GroundFault=on  SwitchTimes=[0.2 0.3]  External=off  SwitchStatus=NaN  FaultResistance=0.001  GroundResistance=0.001  SnubberResistance=1e6  SnubberCapacitance=inf  Measurements=None
  info1 : Subsystem
      settings: OpenFcn="showExample(\"simscapeelectricalsps/LoadFlow29BusNetworkExample\")"
      mask Display: disp('?')
  powergui1 : sps_lib/powergui  Priority=1  SimulationMode=Discrete  SampleTime=75e-6  frequency=60  Iterations=50  frequencyindice=60  Pbase=1e+008  ErrMax=0.0001  UnitsV=kV  UnitsW=MW  buscounter=0  FunctionMessages=off  echomessages=off  EnableUseOfTLC=off  CurrentSourceSwitches=off  DisableSnubberDevices=off  DisableRonSwitches=off  DisableVfSwitches=off  DisplayEquations=off  AutomaticDiscreteSolvers=off  SolverType=Tustin/Backward Euler (TBE)  Interpol=off  ExternalGateDelay=off  methode=off  Ts=100  x0status=blocks  SPID=off  SwTol=0  HookPort=off  NonlinearTolerance=1e-4  nMaxIteration=100  ContinueOnMaxIteration=off  RestoreLinks=warning  ResistiveCurrentMeasurement=off  Frange=[0:2:500]  Ylog=off  Xlog=on  ShowGrid=off  save=off  variable=ZData  structure=0  ZoomFFT=off  StartTime=0.0  cycles=1  DisplayStyle=1  fundamental=60  FreqAxis=off  MaxFrequency=1000  frequencyindicesteady=1  RmsSteady=1  display=off
  send : Outport
  wires:
  receive/1 -> Decoupling_A Send/1
  Regulators1/2(Vf) -> B_5 MTL-5000 MVA1/2
  Decoupling_A Send/1 -> send/1
  Regulators1/1(Pm) -> B_5 MTL-5000 MVA1/1
  B_5 MTL-5000 MVA1/1 -> Regulators1/1(m)
  PSS1/1 -> Subsystem3/1(In1)
  connections:
  QUE1/RConn1 -- North_East Network1/LConn4
  MTL-QUE 5*219km1/RConn2 -- QUE1/LConn2 -- CHM-JCA 2*252km1/RConn2 -- QUE Load and Wind Generation1/LConn2
  Load Flow Bus6/LConn1 -- MTL-QUE 5*219km1/RConn3 -- QUE1/LConn3 -- CHM-JCA 2*252km1/RConn3 -- QUE Load and Wind Generation1/LConn3
  SAG1/RConn2 -- SAG 660Mvar1/LConn2 -- Cs SAG1/LConn2
  5000 MVA 13.8 kV/735 kV2/RConn2 -- Decoupling_A Send/LConn2 -- North-West Network1/RConn2 -- MTL1/LConn2 -- MTL Load1/LConn2
  MTL-QUE 5*219km1/LConn2 -- MTL1/RConn2 -- Three-Phase Fault1/LConn2
  CHM-SAG 117km1/RConn3 -- SAG1/LConn3 -- Load Flow Bus7/LConn1
  CHM-SAG 117km1/LConn3 -- North-West Network1/RConn6 -- Cs CHMS1/LConn3
  QUE1/RConn2 -- North_East Network1/LConn5
  5000 MVA 13.8 kV/735 kV2/LConn3 -- 250 MW1/LConn3 -- B_5 MTL-5000 MVA1/RConn3 -- Load Flow Bus4/LConn1
  SAG1/RConn1 -- SAG 660Mvar1/LConn1 -- Cs SAG1/LConn1
  SAG1/RConn3 -- SAG 660Mvar1/LConn3 -- Cs SAG1/LConn3
  SAG-MIC 247km1/RConn3 -- North_East Network1/LConn3
  Cs CHMS1/RConn2 -- CHM-JCA 2*252km1/LConn2
  CHM-SAG 117km1/LConn2 -- North-West Network1/RConn5 -- Cs CHMS1/LConn2
  CHM-SAG 117km1/LConn1 -- North-West Network1/RConn4 -- Cs CHMS1/LConn1
  Cs SAG1/RConn3 -- SAG-MIC 247km1/LConn3
  SAG-MIC 247km1/RConn2 -- North_East Network1/LConn2
  Cs CHMS1/RConn1 -- CHM-JCA 2*252km1/LConn1
  5000 MVA 13.8 kV/735 kV2/RConn3 -- Decoupling_A Send/LConn1 -- North-West Network1/RConn3 -- MTL1/LConn3 -- MTL Load1/LConn3 -- Load Flow Bus5/LConn1
  MTL Load1/LConn1 -- MTL1/LConn1 -- Decoupling_A Send/LConn3 -- North-West Network1/RConn1 -- 5000 MVA 13.8 kV/735 kV2/RConn1
  MTL-QUE 5*219km1/LConn1 -- MTL1/RConn1 -- Three-Phase Fault1/LConn1
  Cs SAG1/RConn1 -- SAG-MIC 247km1/LConn1
  MTL-QUE 5*219km1/RConn1 -- QUE1/LConn1 -- CHM-JCA 2*252km1/RConn1 -- QUE Load and Wind Generation1/LConn1
  Cs CHMS1/RConn3 -- CHM-JCA 2*252km1/LConn3
  Cs SAG1/RConn2 -- SAG-MIC 247km1/LConn2
  SAG1/LConn2 -- CHM-SAG 117km1/RConn2
  QUE1/RConn3 -- North_East Network1/LConn6
  SAG1/LConn1 -- CHM-SAG 117km1/RConn1
  SAG-MIC 247km1/RConn1 -- North_East Network1/LConn1
  250 MW1/LConn1 -- 5000 MVA 13.8 kV/735 kV2/LConn1 -- B_5 MTL-5000 MVA1/RConn1
  250 MW1/LConn2 -- 5000 MVA 13.8 kV/735 kV2/LConn2 -- B_5 MTL-5000 MVA1/RConn2
  MTL-QUE 5*219km1/LConn3 -- MTL1/RConn3 -- Three-Phase Fault1/LConn3

== system LoadFlow58BusNetwork_2024/Subsystem/Cs CHMS1 ==
  note: B
  Ca : spsSeriesRLCBranchLib/Series RLC Branch  LConnTagsString=__new0  RConnTagsString=__new0  BranchType=C  Resistance=1.0  Inductance=1.0  SetiL0=off  InitialCurrent=0  Capacitance=Cs  Setx0=off  InitialVoltage=0  Measurements=None
  Cb : spsSeriesRLCBranchLib/Series RLC Branch  LConnTagsString=__new0  RConnTagsString=__new0  BranchType=C  Resistance=1.0  Inductance=1.0  SetiL0=off  InitialCurrent=0  Capacitance=Cs  Setx0=off  InitialVoltage=0  Measurements=None
  Cc : spsSeriesRLCBranchLib/Series RLC Branch  LConnTagsString=__new0  RConnTagsString=__new0  BranchType=C  Resistance=1.0  Inductance=1.0  SetiL0=off  InitialCurrent=0  Capacitance=Cs  Setx0=off  InitialVoltage=0  Measurements=None
  A : PMIOPort  Side=Left
  B : PMIOPort  Port=2  Side=Left
  C : PMIOPort  Port=3  Side=Left
  "A " : PMIOPort  Port=4  Side=Right
  "B " : PMIOPort  Port=5  Side=Right
  "C " : PMIOPort  Port=6  Side=Right
  connections:
  Cc/RConn1 -- "C "/RConn1
  C/RConn1 -- Cc/LConn1
  Cb/RConn1 -- "B "/RConn1
  B/RConn1 -- Cb/LConn1
  Ca/RConn1 -- "A "/RConn1
  A/RConn1 -- Ca/LConn1

== system LoadFlow58BusNetwork_2024/Subsystem/Cs SAG1 ==
  note: B
  Ca : spsSeriesRLCBranchLib/Series RLC Branch  LConnTagsString=__new0  RConnTagsString=__new0  BranchType=C  Resistance=1.0  Inductance=1.0  SetiL0=off  InitialCurrent=0  Capacitance=Cs  Setx0=off  InitialVoltage=0  Measurements=None
  Cb : spsSeriesRLCBranchLib/Series RLC Branch  LConnTagsString=__new0  RConnTagsString=__new0  BranchType=C  Resistance=1.0  Inductance=1.0  SetiL0=off  InitialCurrent=0  Capacitance=Cs  Setx0=off  InitialVoltage=0  Measurements=None
  Cc : spsSeriesRLCBranchLib/Series RLC Branch  LConnTagsString=__new0  RConnTagsString=__new0  BranchType=C  Resistance=1.0  Inductance=1.0  SetiL0=off  InitialCurrent=0  Capacitance=Cs  Setx0=off  InitialVoltage=0  Measurements=None
  A : PMIOPort  Side=Left
  B : PMIOPort  Port=2  Side=Left
  C : PMIOPort  Port=3  Side=Left
  "A " : PMIOPort  Port=4  Side=Right
  "B " : PMIOPort  Port=5  Side=Right
  "C " : PMIOPort  Port=6  Side=Right
  connections:
  A/RConn1 -- Ca/LConn1
  Ca/RConn1 -- "A "/RConn1
  B/RConn1 -- Cb/LConn1
  Cb/RConn1 -- "B "/RConn1
  C/RConn1 -- Cc/LConn1
  Cc/RConn1 -- "C "/RConn1

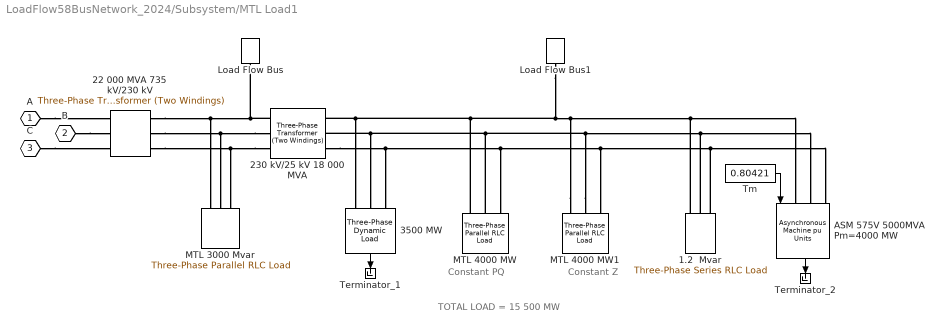
== system LoadFlow58BusNetwork_2024/Subsystem/MTL Load1 ==
  note: Constant PQ
  note: Constant Z
  note: TOTAL LOAD = 15 500 MW
  1.2  Mvar : spsThreePhaseSeriesRLCLoadLib/Three-Phase Series RLC Load  LConnTagsString=A|B|C  Configuration=Y (grounded)  NominalVoltage=25e3  Vabc=[1e3 1e3 1e3]  Vabcp=[1e3 1e3 1e3]  NominalFrequency=60  UnbalancedPower=off  ActivePower=2000e6/50  InductivePower=0  CapacitivePower=2000e6  Pabc=[10e3 9e3 11e3]  QLabc=[100 90 110]  QCabc=[100 90 110]  Pabcp=[10e3 9e3 11e3]  QLabcp=[100 90 110]  QCabcp=[100 90 110]  Measurements=None  LoadType=constant Z
  22 000 MVA 735 kV/230 kV : spsThreePhaseTransformerTwoWindingsLib/Three-Phase Transformer (Two Windings)  Winding1Connection=Yg  Winding2Connection=Delta (D1)  CoreType=Three single-phase transformers  SetSaturation=off  Hysteresis=off  DataFile='basic_model'  SetInitialFlux=off  Measurements=None  UNITS=pu  NominalPower=[ 22000e6 60 ]  Winding1="[ 735e3 0.002  0.12]"  Winding2=[230e3 0.002 0]  Rm=500  Lm=500  L0=0.5  Saturation="[ 0,0  ;  0.005,1.2  ;  1.0,1.4 ]"  InitialFluxes=[ 0.8 , -0.8 , 0.7 ]  BreakLoop=off  DiscreteSolver=Trapezoidal iterative  DataType=off  TransfoNumber=0
  230 kV/25 kV 18 000 MVA : spsThreePhaseTransformerTwoWindingsLib/Three-Phase Transformer (Two Windings)  Winding1Connection=Yg  Winding2Connection=Delta (D1)  CoreType=Three single-phase transformers  SetSaturation=off  Hysteresis=off  DataFile='basic_model'  SetInitialFlux=off  Measurements=None  UNITS=pu  NominalPower=[18000e6 60 ]  Winding1="[ 230e3  0.08/30   0.08 ]"  Winding2="[ 25e3  0.08/30  0.08]"  Rm=500  Lm=500  L0=0.5  Saturation="[ 0,0  ;  0.005,1.2  ;  1.0,1.4 ]"  InitialFluxes=[ 0.8 , -0.8 , 0.7 ]  BreakLoop=off  DiscreteSolver=Trapezoidal iterative  DataType=off  TransfoNumber=0
  3500 MW : spsThreePhaseDynamicLoadLib/Three-Phase Dynamic Load  NominalVoltage=[ 25e3 60 ]  ActiveReactivePowers=[3.5e+09 4.44089e-08]  PositiveSequence=[0.991615 -96.3945]  ExternalControl=off  NpNq="[1.5  2.5]"  TimeConstants="[0  0  0  0]"  MinimumVoltage=0.7  Tfilter=1e-4  LoadFlowParameters=[4,0,0,0,0]
      settings: LibrarySourceBlock=|
      | sps_lib/Passives/Three-Phase
      | Dynamic Load
  ASM 575V 5000MVA Pm=4000 MW : spsAsynchronousMachinepuUnitsLib/Asynchronous Machine pu Units  RotorType=Squirrel-cage  PresetModel=No  MechanicalLoad=Torque Tm  ShowDetailedParameters=on  ReferenceFrame=Rotor  Units=pu  MeasurementBus=off  NominalParameters="[5000e6 25e3  60]"  VoltageRatio=1  Stator=[0.01117 0.04832]  Rotor=[0.006 0.04832]  Cage1=[0.01909 0.0397]  Cage2=[0.01909 0.0397]  Lm=2.424  Mechanical="[1  0   2]"  PolePairs=2  InitialConditions=[0.00523668 0 0.941796 0.941796 0.941796 -125.733 -245.733 -5.73298]  SimulateSaturation=off  Saturation="[0.212,0.4201,0.8125,1.0979,1.4799,2.2457,3.2586,4.5763,6.4763 ;   0.5,0.7,0.9,1,1.1,1.2 ,1.3,1.4,1.5]"  LoadFlowParameters=0  TsPowergui=0  TsBlock=-1  IterativeModel=Trapezoidal non iterative  IterativeDiscreteModel=Trapezoidal non iterative  Pmec=4000000000
      settings: LibrarySourceBlock=|
      | sps_lib/Electrical Machines/Asynchronous Machine
      | pu Units
  Load Flow Bus : spsLoadFlowBusLib/Load Flow Bus  LConnTagsString=a  Phases=single  Connectors=on one side  ID=MTL2  Vbase=230e3  Vref=1  Vangle=0  VLF=1.009  VLFb=1  VLFc=1  angleLF=-58.45  angleLFb=0  angleLFc=0
      settings: AttributesFormatString=%<ID>\n%<Vbase>V\n%<VLF>pu\n%<angleLF>deg.
  Load Flow Bus1 : spsLoadFlowBusLib/Load Flow Bus  LConnTagsString=a  Phases=single  Connectors=on one side  ID=MTL_25  Vbase=25e3  Vref=1  Vangle=0  VLF=0.9916  VLFb=1  VLFc=1  angleLF=-96.39  angleLFb=0  angleLFc=0
      settings: AttributesFormatString=%<ID>\n%<Vbase>V\n%<VLF>pu\n%<angleLF>deg.
  MTL 3000 Mvar : spsThreePhaseParallelRLCLoadLib/Three-Phase Parallel RLC Load  LConnTagsString=A|B|C  Configuration=Y (grounded)  NominalVoltage=230e3  Vabc=[1e3 1e3 1e3]  Vabcp=[1e3 1e3 1e3]  NominalFrequency=60  UnbalancedPower=off  ActivePower=0  InductivePower=0  CapacitivePower=3000e6  Pabc=[10e3 9e3 11e3]  QLabc=[100 90 110]  QCabc=[100 90 110]  Pabcp=[10e3 9e3 11e3]  QLabcp=[100 90 110]  QCabcp=[100 90 110]  Measurements=None  LoadType=constant Z
  MTL 4000 MW : spsThreePhaseParallelRLCLoadLib/Three-Phase Parallel RLC Load  LConnTagsString=A|B|C  Configuration=Y (grounded)  NominalVoltage=(25000)*0.991615  Vabc=[1e3 1e3 1e3]  Vabcp=[1e3 1e3 1e3]  NominalFrequency=60  UnbalancedPower=off  ActivePower=4000000000  InductivePower=0  CapacitivePower=0  Pabc=[10e3 9e3 11e3]  QLabc=[100 90 110]  QCabc=[100 90 110]  Pabcp=[10e3 9e3 11e3]  QLabcp=[100 90 110]  QCabcp=[100 90 110]  Measurements=None  LoadType=constant PQ
  MTL 4000 MW1 : spsThreePhaseParallelRLCLoadLib/Three-Phase Parallel RLC Load  LConnTagsString=A|B|C  Configuration=Y (grounded)  NominalVoltage=25e3  Vabc=[1e3 1e3 1e3]  Vabcp=[1e3 1e3 1e3]  NominalFrequency=60  UnbalancedPower=off  ActivePower=4000000000  InductivePower=0  CapacitivePower=0  Pabc=[10e3 9e3 11e3]  QLabc=[100 90 110]  QCabc=[100 90 110]  Pabcp=[10e3 9e3 11e3]  QLabcp=[100 90 110]  QCabcp=[100 90 110]  Measurements=None  LoadType=constant Z
  Terminator_1 : Terminator
  Terminator_2 : Terminator
  Tm : Constant  Value=0.80421
  A : PMIOPort  Side=Left
  B : PMIOPort  Port=2  Side=Left
  C : PMIOPort  Port=3  Side=Left
  wires:
  Tm/1 -> ASM 575V 5000MVA Pm=4000 MW/1
  3500 MW/1 -> Terminator_1/1
  ASM 575V 5000MVA Pm=4000 MW/1 -> Terminator_2/1
  connections:
  A/RConn1 -- 22 000 MVA 735 kV/230 kV/LConn1
  B/RConn1 -- 22 000 MVA 735 kV/230 kV/LConn2
  C/RConn1 -- 22 000 MVA 735 kV/230 kV/LConn3
  230 kV/25 kV 18 000 MVA/LConn1 -- Load Flow Bus/LConn1 -- 22 000 MVA 735 kV/230 kV/RConn1 -- MTL 3000 Mvar/LConn1
  230 kV/25 kV 18 000 MVA/LConn2 -- 22 000 MVA 735 kV/230 kV/RConn2 -- MTL 3000 Mvar/LConn2
  230 kV/25 kV 18 000 MVA/LConn3 -- 22 000 MVA 735 kV/230 kV/RConn3 -- MTL 3000 Mvar/LConn3
  MTL 4000 MW1/LConn1 -- Load Flow Bus1/LConn1 -- MTL 4000 MW/LConn1 -- 230 kV/25 kV 18 000 MVA/RConn1 -- 3500 MW/LConn1 -- ASM 575V 5000MVA Pm=4000 MW/LConn1 -- 1.2  Mvar/LConn1
  MTL 4000 MW1/LConn2 -- MTL 4000 MW/LConn2 -- 230 kV/25 kV 18 000 MVA/RConn2 -- 3500 MW/LConn2 -- ASM 575V 5000MVA Pm=4000 MW/LConn2 -- 1.2  Mvar/LConn2
  230 kV/25 kV 18 000 MVA/RConn3 -- ASM 575V 5000MVA Pm=4000 MW/LConn3 -- 1.2  Mvar/LConn3 -- MTL 4000 MW1/LConn3 -- MTL 4000 MW/LConn3 -- 3500 MW/LConn3
